simulink model "PrimeiraOrdem"  (R2015a)
settings: Solver=ode45  StartTime=0.0  StopTime=10.0  RelTol=1e-3
libraries: simulink x1
settings Model: Creator=user  LastModifiedBy=user
settings SolverCC: ZeroCrossAlgorithm=Adaptive

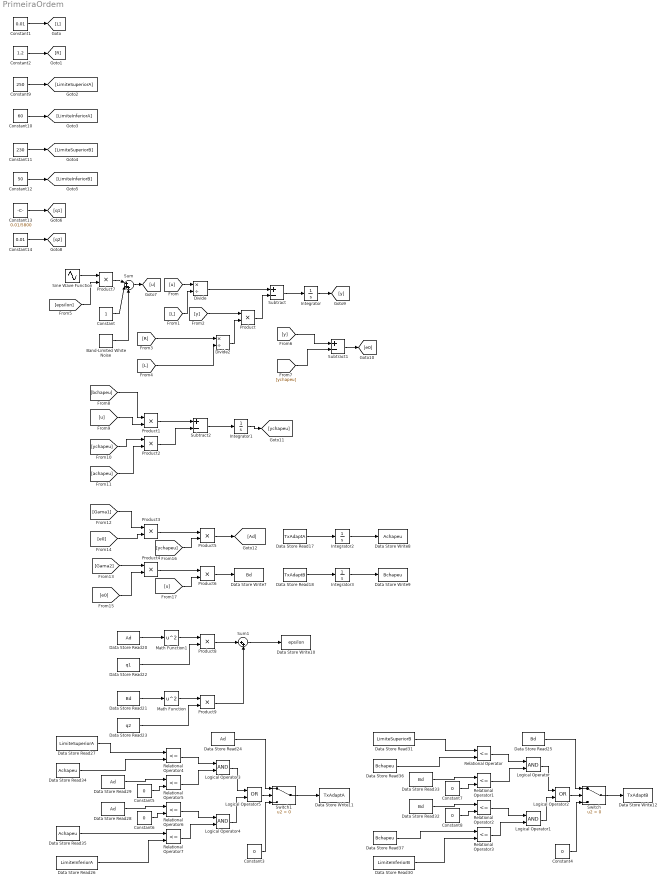
== system PrimeiraOrdem ==
  Band-Limited White Noise : simulink/Sources/Band-Limited White Noise  Cov=[0.1]  Ts=0.1  seed=[23341]
  Constant : Constant
  Constant1 : Constant  Value=0.01
  Constant10 : Constant  Value=60
  Constant11 : Constant  Value=230
  Constant12 : Constant  Value=50
  Constant13 : Constant  Value=0.01/5800
  Constant14 : Constant  Value=0.01
  Constant2 : Constant  Value=1.2
  Constant{3..8} (6 alike) : Constant  Value=0
  Constant9 : Constant  Value=250
  Data Store Read17 : DataStoreRead  DataStoreName=TxAdaptA
  Data Store Read18 : DataStoreRead  DataStoreName=TxAdaptB
  Data Store Read{20,24,28..29} (4 alike) : DataStoreRead  DataStoreName=Ad
  Data Store Read{21,25,32..33} (4 alike) : DataStoreRead  DataStoreName=Bd
  Data Store Read22 : DataStoreRead  DataStoreName=q1
  Data Store Read23 : DataStoreRead  DataStoreName=q2
  Data Store Read26 : DataStoreRead  DataStoreName=LimiteInferiorA
  Data Store Read27 : DataStoreRead  DataStoreName=LimiteSuperiorA
  Data Store Read30 : DataStoreRead  DataStoreName=LimiteInferiorB
  Data Store Read31 : DataStoreRead  DataStoreName=LimiteSuperiorB
  Data Store Read34 : DataStoreRead  DataStoreName=Achapeu
  Data Store Read35 : DataStoreRead  DataStoreName=Achapeu
  Data Store Read36 : DataStoreRead  DataStoreName=Bchapeu
  Data Store Read37 : DataStoreRead  DataStoreName=Bchapeu
  Data Store Write10 : DataStoreWrite  DataStoreName=epsilon
  Data Store Write11 : DataStoreWrite  DataStoreName=TxAdaptA
  Data Store Write12 : DataStoreWrite  DataStoreName=TxAdaptB
  Data Store Write7 : DataStoreWrite  DataStoreName=Bd
  Data Store Write8 : DataStoreWrite  DataStoreName=Achapeu
  Data Store Write9 : DataStoreWrite  DataStoreName=Bchapeu
  Divide : Product  Inputs=*/
  Divide2 : Product  Inputs=*/
  Integrator{,1..3} (4 alike) : Integrator
  Logical Operator{,1,3..4} (4 alike) : Logic  AllPortsSameDT=off  OutDataTypeStr=boolean
  Logical Operator2 : Logic  Operator=OR  AllPortsSameDT=off  OutDataTypeStr=boolean
  Logical Operator5 : Logic  Operator=OR  AllPortsSameDT=off  OutDataTypeStr=boolean
  Math Function : Math  Operator=square  SaturateOnIntegerOverflow=on
  Math Function1 : Math  Operator=square  SaturateOnIntegerOverflow=on
  Product{,1..9} (10 alike) : Product
  Relational Operator{,1..7} (8 alike) : RelationalOperator  Operator=<=  OutDataTypeStr=boolean
  Sine Wave Function : Sin  SampleTime=0
  Subtract : Sum  Inputs=+-
  Subtract1 : Sum  Inputs=+-
  Subtract2 : Sum  Inputs=+-
  Sum : Sum  Inputs=|+++
  Sum1 : Sum  Inputs=|++
  Switch : Switch  Criteria=u2 > Threshold
  Switch1 : Switch  Criteria=u2 > Threshold
  wires:
  Constant/1 -> Sum/2
  Band-Limited White Noise/1 -> Sum/3
  [L] -> Divide/2
  Divide2/1 -> Product/2
  [L] -> Divide2/2
  [R] -> Divide2/1
  Product/1 -> Subtract/2
  Divide/1 -> Subtract/1
  Subtract/1 -> Integrator/1
  Integrator/1 -> [y]
  [y] -> Product/1
  Sum/1 -> [u]
  [u] -> Divide/1
  [y] -> Subtract1/1
  [ychapeu] -> Subtract1/2
  Subtract1/1 -> [e0]
  Constant1/1 -> [L]
  Constant2/1 -> [R]
  Product1/1 -> Subtract2/1
  Subtract2/1 -> Integrator1/1
  Product2/1 -> Subtract2/2
  [achapeu] -> Product2/2
  [ychapeu] -> Product2/1
  [u] -> Product1/2
  [bchapeu] -> Product1/1
  Integrator1/1 -> [ychapeu]
  [e0] -> Product3/2
  [Gama1] -> Product3/1
  [Gama2] -> Product4/1
  [e0] -> Product4/2
  Product4/1 -> Product6/1
  Product3/1 -> Product5/1
  [ychapeu] -> Product5/2
  [u] -> Product6/2
  Product6/1 -> Data Store Write7/1
  Product5/1 -> [Ad]
  Data Store Read17/1 -> Integrator2/1
  Data Store Read18/1 -> Integrator3/1
  Integrator3/1 -> Data Store Write9/1
  Integrator2/1 -> Data Store Write8/1
  Product7/1 -> Sum/1
  Sine Wave Function/1 -> Product7/1
  [epsilon] -> Product7/2
  Data Store Read21/1 -> Math Function/1
  Data Store Read20/1 -> Math Function1/1
  Math Function1/1 -> Product8/1
  Math Function/1 -> Product9/1
  Data Store Read22/1 -> Product8/2
  Data Store Read23/1 -> Product9/2
  Product9/1 -> Sum1/2
  Product8/1 -> Sum1/1
  Sum1/1 -> Data Store Write10/1
  Relational Operator2/1 -> Logical Operator1/1
  Relational Operator3/1 -> Logical Operator1/2
  Relational Operator1/1 -> Logical Operator/2
  Relational Operator/1 -> Logical Operator/1
  Logical Operator/1 -> Logical Operator2/1
  Logical Operator1/1 -> Logical Operator2/2
  Relational Operator6/1 -> Logical Operator4/1
  Relational Operator7/1 -> Logical Operator4/2
  Relational Operator5/1 -> Logical Operator3/2
  Relational Operator4/1 -> Logical Operator3/1
  Logical Operator3/1 -> Logical Operator5/1
  Logical Operator4/1 -> Logical Operator5/2
  Logical Operator2/1 -> Switch/2
  Logical Operator5/1 -> Switch1/2
  Data Store Read24/1 -> Switch1/1
  Data Store Read25/1 -> Switch/1
  Constant3/1 -> Switch1/3
  Constant4/1 -> Switch/3
  Switch1/1 -> Data Store Write11/1
  Switch/1 -> Data Store Write12/1
  Data Store Read27/1 -> Relational Operator4/1
  Data Store Read26/1 -> Relational Operator7/2
  Constant6/1 -> Relational Operator6/2
  Constant5/1 -> Relational Operator5/2
  Data Store Read28/1 -> Relational Operator6/1
  Data Store Read29/1 -> Relational Operator5/1
  Data Store Read31/1 -> Relational Operator/1
  Data Store Read30/1 -> Relational Operator3/2
  Data Store Read32/1 -> Relational Operator2/1
  Data Store Read33/1 -> Relational Operator1/1
  Constant8/1 -> Relational Operator2/2
  Constant7/1 -> Relational Operator1/2
  Constant9/1 -> [LimiteSuperiorA]
  Constant10/1 -> [LimiteInferiorA]
  Constant11/1 -> [LimiteSuperiorB]
  Constant12/1 -> [LimiteInferiorB]
  Data Store Read35/1 -> Relational Operator7/1
  Data Store Read34/1 -> Relational Operator4/2
  Data Store Read36/1 -> Relational Operator/2
  Data Store Read37/1 -> Relational Operator3/1
  Constant13/1 -> [q1]
  Constant14/1 -> [q2]
